simulink library "motor_lib"  (Simulink 8.1)
settings: Solver=ode45  StartTime=0.0  StopTime=10.0  RelTol=1e-3
undefined symbols (not defined in the file): Ts
libraries: powerlib x2, Motor_InductionMachine_lib x1, breaker_lib x1
settings Model: Creator=re25624  LastModifiedBy=ed12083

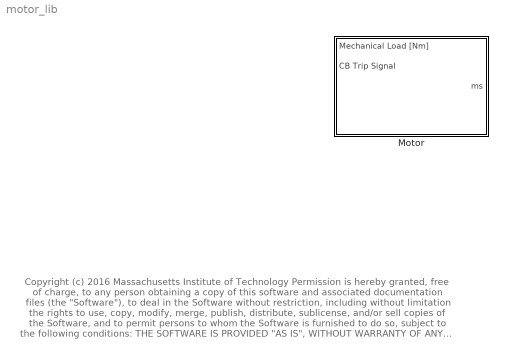
== system motor_lib ==
  note: Copyright (c) 2016 Massachusetts Institute of Technology
      | Permission is hereby granted, free of charge, to any person obtaining a copy of this software and associated documentation files (the "Software"), to deal
      | in the Software without restriction, including without limitation the rights to use, copy, modify, merge, publish, distribute, sublicense, and/or sell copies of the
      | Software, and to permit persons to whom the Software is furnished to do so, subject to the following conditions:
      |
      | THE SOFTWARE IS PROVIDED "AS IS", WITHOUT WARRANTY OF ANY KIND, EXPRESS OR IMPLIED, INCLUDING BUT NOT LIMITED TO THE
      | WARRANTIES OF MERCHANTABILITY, FITNESS FOR A PARTICULAR PURPOSE AND NONINFRINGEMENT. IN NO EVENT SHALL THE AUTHORS
      | OR COPYRIGHT HOLDERS BE LIABLE FOR ANY CLAIM, DAMAGES OR OTHER LIABILITY, WHETHER IN AN ACTION OF CONTRACT, TORT OR
      | OTHERWISE, ARISING FROM, OUT OF OR IN CONNECTION WITH THE SOFTWARE OR THE USE OR OTHER DEALINGS IN THE SOFTWARE.
  Motor : Subsystem

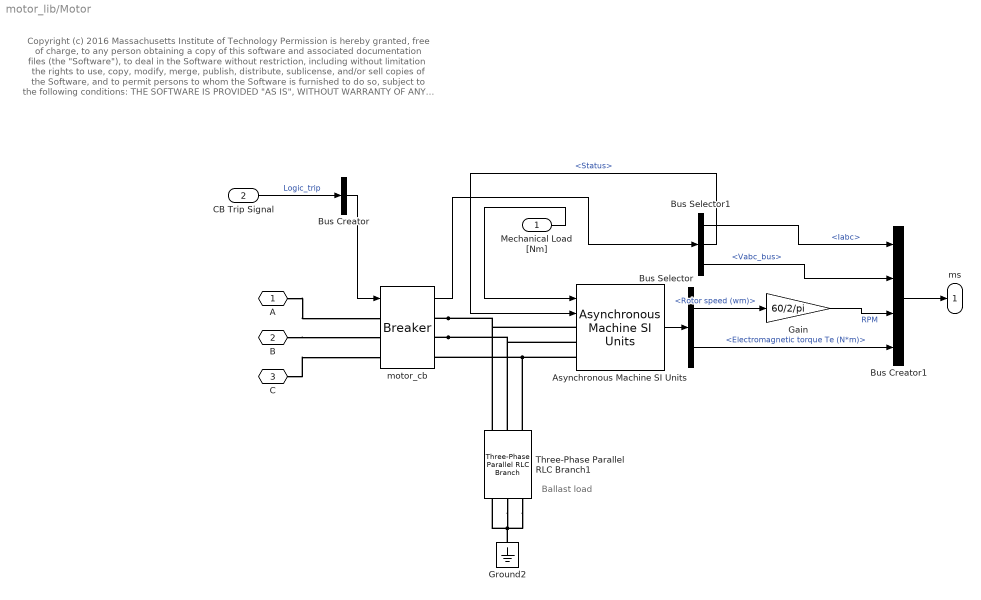
== system motor_lib/Motor ==
  note: Ballast load
  note: Copyright (c) 2016 Massachusetts Institute of Technology
      | Permission is hereby granted, free of charge, to any person obtaining a copy of this software and associated documentation files (the "Software"), to deal
      | in the Software without restriction, including without limitation the rights to use, copy, modify, merge, publish, distribute, sublicense, and/or sell copies of the
      | Software, and to permit persons to whom the Software is furnished to do so, subject to the following conditions:
      |
      | THE SOFTWARE IS PROVIDED "AS IS", WITHOUT WARRANTY OF ANY KIND, EXPRESS OR IMPLIED, INCLUDING BUT NOT LIMITED TO THE
      | WARRANTIES OF MERCHANTABILITY, FITNESS FOR A PARTICULAR PURPOSE AND NONINFRINGEMENT. IN NO EVENT SHALL THE AUTHORS
      | OR COPYRIGHT HOLDERS BE LIABLE FOR ANY CLAIM, DAMAGES OR OTHER LIABILITY, WHETHER IN AN ACTION OF CONTRACT, TORT OR
      | OTHERWISE, ARISING FROM, OUT OF OR IN CONNECTION WITH THE SOFTWARE OR THE USE OR OTHER DEALINGS IN THE SOFTWARE.
  Mechanical Load [Nm] : Inport
  CB Trip Signal : Inport  Port=2
  Asynchronous Machine SI Units : Motor_InductionMachine_lib/Asynchronous Machine SI Units  PresetModel=No  MechanicalLoad=Torque Tm  ShowDetailedParameters=on  RotorType=Squirrel-cage  ReferenceFrame=Stationary  NominalParameters=[ 136700/.92/.93, 480, 60 ]  Stator=[ 0.029 0.226/377/1.5]  Rotor=[ 0.022*3 0.226/377/1.5]  Cage1=[ 0.022 0.226/377]  Cage2=[ 0.022 0.226/377]  Lm=13.04/377  Mechanical="[ 63.87 0  2 ]"  PolePairs=2  InitialConditions=[1 0 0 0 0 0 0 0]  Units=SI  LoadFlowParameters=1492000  SimulateSaturation=off  Saturation=[14.03593122, 27.81365428, 53.79336849, 72.68890987, 97.98006896, 148.6815601, 215.7428561, 302.9841135, 420.4778367 ; 230, 322, 414, 460, 506, 552, 598, 644, 690]  TsPowergui=0  TsBlock=-1  IterativeModel=Trapezoidal non iterative  Pmec=0
      settings: AttributesFormatString=\n
  Bus Creator : BusCreator  Inputs=1
  Bus Creator1 : BusCreator
  Bus Selector : BusSelector  OutputSignals=Mechanical.Rotor speed (wm),Mechanical.Electromagnetic torque Te (N*m)
  Bus Selector1 : BusSelector  OutputSignals=Iabc,Status,Vabc_bus
  Gain : Gain  Gain=60/2/pi
  Ground2 : powerlib/Elements/Ground  LConnTagsString=a
  Three-Phase Parallel RLC Branch1 : powerlib/Elements/Three-Phase Parallel RLC Branch  LConnTagsString=A|B|C  RConnTagsString=A|B|C  BranchType=RC  Resistance=1e6  Inductance=inf  Capacitance=10e-6  Measurements=None
  motor_cb : breaker_lib/Breaker  Ts=Ts
  A : PMIOPort  Port=1  Side=Left
  B : PMIOPort  Port=2  Side=Left
  C : PMIOPort  Port=3  Side=Left
  ms : Outport
  wires:
  Bus Selector1/2 -> Asynchronous Machine SI Units/2  "<Status>"
  Bus Selector1/1 -> Bus Creator1/1  "<Iabc>"
  Bus Selector1/3 -> Bus Creator1/2  "<Vabc_bus>"
  Bus Creator1/1 -> ms/1
  CB Trip Signal/1 -> Bus Creator/1  "Logic_trip"
  Bus Creator/1 -> motor_cb/1
  Mechanical Load [Nm]/1 -> Asynchronous Machine SI Units/1
  Asynchronous Machine SI Units/1 -> Bus Selector/1
  Bus Selector/1 -> Gain/1  "<Rotor speed (wm)>"
  Bus Selector/2 -> Bus Creator1/4  "<Electromagnetic torque Te (N*m)>"
  Gain/1 -> Bus Creator1/3  "RPM"
  motor_cb/1 -> Bus Selector1/1
  connections:
  motor_cb/RConn1 -- Three-Phase Parallel RLC Branch1/RConn1 -- Asynchronous Machine SI Units/LConn1
  motor_cb/RConn2 -- Three-Phase Parallel RLC Branch1/RConn2 -- Asynchronous Machine SI Units/LConn2
  Asynchronous Machine SI Units/LConn3 -- motor_cb/RConn3 -- Three-Phase Parallel RLC Branch1/RConn3
  Three-Phase Parallel RLC Branch1/LConn2 -- Three-Phase Parallel RLC Branch1/LConn3 -- Ground2/LConn1 -- Three-Phase Parallel RLC Branch1/LConn1
  A/RConn1 -- motor_cb/LConn1
  B/RConn1 -- motor_cb/LConn2
  C/RConn1 -- motor_cb/LConn3
